simulink library "eltreclib"  (R2017a)
settings: Solver=VariableStepAuto  StartTime=0.0  StopTime=10.0  RelTol=1e-3
undefined symbols (not defined in the file or in its folder): Jr
libraries: powerlib x79
settings Model: Creator=mayartmal  LastModifiedBy=mayartmal

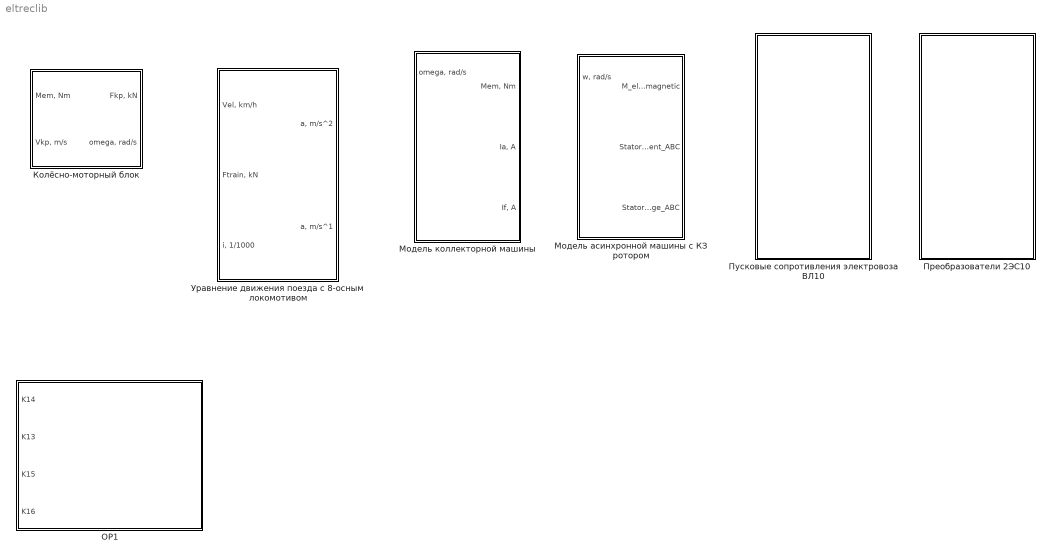
== system eltreclib ==
  OP1 : Subsystem
      mask DialogControl DescTextVar Prompt: Резисторы ослабления поля
  Колёсно-моторный блок : Subsystem  mask{Db=0, mu=0}
      mask prompts: Db "Диаметр бандажа, м"; mu "Передаточное отношение редуктора"
      mask DialogControl DescTextVar Prompt: Здесь можно вписать описание, формулы и другую полезную информацию
  Модель асинхронной машины с КЗ ротором : Subsystem  mask(Модель асинхронной машины){f_nominal=50, Rs=0.0472, ls=0.0003883, Rr=0.0392, lr=0.0005399, Lm=0.011, Zp=2}
      mask prompts: f_nominal "Номинальная частота, Гц"; Rs "Активное сопротивление статора, Ом"; ls "Индуктивность статора, Гн"; Rr "Активное сопротивление ротора, Ом"; lr "Индуктивность ротора, Гн"; Lm "Взаимная индуктивность, Гн"; Zp "Число пар полюсов"
      mask help: Модель учитывает только электрические параметры схемы замещения и не учитывает механику
      mask init:
      | Ls = ls + Lm;
      | Lr = lr + Lm;
      | Kr = Lm / Lr;
      | Ks = Lm / Ls;
      | sigma = 1 - (Lm ^ 2) / (Ls * Lr);
      | w_s = (2 * pi * f_nominal) / Zp;
  Модель коллекторной машины : Subsystem  mask{Rf=0, Lf=0, Ra=0, La=0, Ce=0, Cm=0, A=0, B=0}
      mask prompts: Rf "Активное сопротивление обмотки возбуждения, Ом"; Lf "Индуктивность обмотки возбуждения, Гн"; Ra "Активное сопротивление обмотки якоря, Ом"; La "Индуктивность обмотки якоря, Гн"; Ce "Константа Ce"; Cm "Константа Cm"; A "Коэффициент A"; B "Коэффициент B"
      mask DialogControl DescTextVar Prompt: Здесь можно вписать описание, формулы и другую полезную информацию
  Преобразователи 2ЭС10 : Subsystem
  Пусковые сопротивления электровоза ВЛ10 : Subsystem
  Уравнение движения поезда c 8-осным локомотивом : Subsystem  mask{a0=16, a1=0.176, a2=0.0079, P=112}
      mask prompts: a0 "Коэффициент a0"; a1 "Коэффициент a1"; a2 "Коэффициент a2"; P "Масса поезда, т"
      mask DialogControl DescTextVar Prompt: Здесь можно вписать описание, формулы и другую полезную информацию

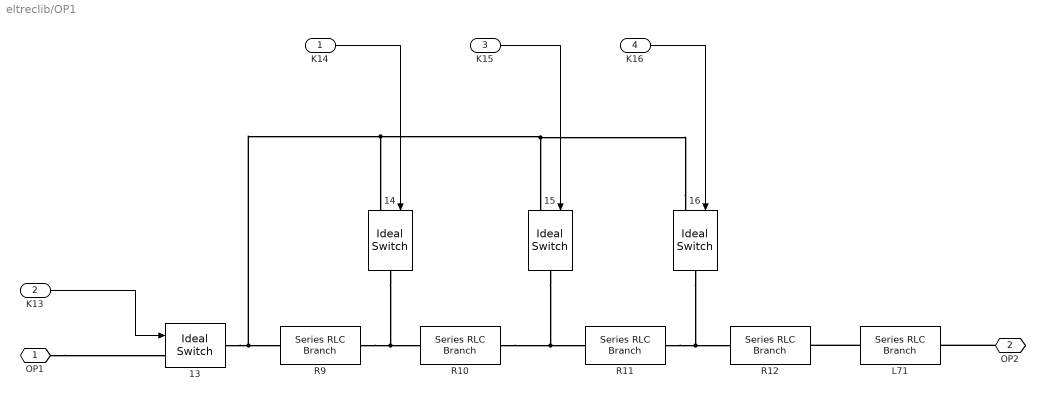
== system eltreclib/OP1 ==
  K14 : Inport
  K13 : Inport  Port=2
  K15 : Inport  Port=3
  K16 : Inport  Port=4
  {13..16} (4 alike) : powerlib/Power Electronics/Ideal Switch  Ron=0.001  Lon=0  IC=0  Rs=1e6  Cs=inf  Measurements=off
  L71 : powerlib/Elements/Series RLC Branch  LConnTagsString=__new0  RConnTagsString=__new0  BranchType=RL  Resistance=0.0236  Inductance=4.5e-3  SetiL0=off  InitialCurrent=0  Capacitance=1e-6  Setx0=off  InitialVoltage=0  Measurements=None
  R10 : powerlib/Elements/Series RLC Branch  LConnTagsString=__new0  RConnTagsString=__new0  BranchType=R  Resistance=0.04  Inductance=1e-3  SetiL0=off  InitialCurrent=0  Capacitance=1e-6  Setx0=off  InitialVoltage=0  Measurements=None
  R11 : powerlib/Elements/Series RLC Branch  LConnTagsString=__new0  RConnTagsString=__new0  BranchType=R  Resistance=0.0222  Inductance=1e-3  SetiL0=off  InitialCurrent=0  Capacitance=1e-6  Setx0=off  InitialVoltage=0  Measurements=None
  R12 : powerlib/Elements/Series RLC Branch  LConnTagsString=__new0  RConnTagsString=__new0  BranchType=R  Resistance=0.01  Inductance=1e-3  SetiL0=off  InitialCurrent=0  Capacitance=1e-6  Setx0=off  InitialVoltage=0  Measurements=None
  R9 : powerlib/Elements/Series RLC Branch  LConnTagsString=__new0  RConnTagsString=__new0  BranchType=R  Resistance=0.1407  Inductance=1e-3  SetiL0=off  InitialCurrent=0  Capacitance=1e-6  Setx0=off  InitialVoltage=0  Measurements=None
  OP1 : PMIOPort  Port=1  Side=Right
  OP2 : PMIOPort  Port=2  Side=Right
  wires:
  K16/1 -> 16/1
  K15/1 -> 15/1
  K13/1 -> 13/1
  K14/1 -> 14/1
  connections:
  OP2/RConn1 -- L71/RConn1
  L71/LConn1 -- R12/RConn1
  OP1/RConn1 -- 13/LConn1
  16/LConn1 -- 14/LConn1 -- 13/RConn1 -- R9/LConn1 -- 15/LConn1
  16/RConn1 -- R11/RConn1 -- R12/LConn1
  15/RConn1 -- R10/RConn1 -- R11/LConn1
  14/RConn1 -- R9/RConn1 -- R10/LConn1

== system eltreclib/Колёсно-моторный блок ==
  "Mem, Nm" : Inport
  "Vkp, m/s" : Inport  Port=2
  Gain : Gain  Gain=mu
  Gain1 : Gain  Gain=2/Db
  Gain2 : Gain  Gain=0.001
  Gain5 : Gain  Gain=2/Db
  Gain6 : Gain  Gain=mu
  "Fkp, kN" : Outport
  "omega, rad/s" : Outport  Port=2
  wires:
  Gain/1 -> Gain1/1  "Mkp, Nm"
  "Mem, Nm"/1 -> Gain/1
  Gain1/1 -> Gain2/1  "Fkp, N"
  Gain5/1 -> Gain6/1
  "Vkp, m/s"/1 -> Gain5/1
  Gain6/1 -> "omega, rad/s"/1
  Gain2/1 -> "Fkp, kN"/1

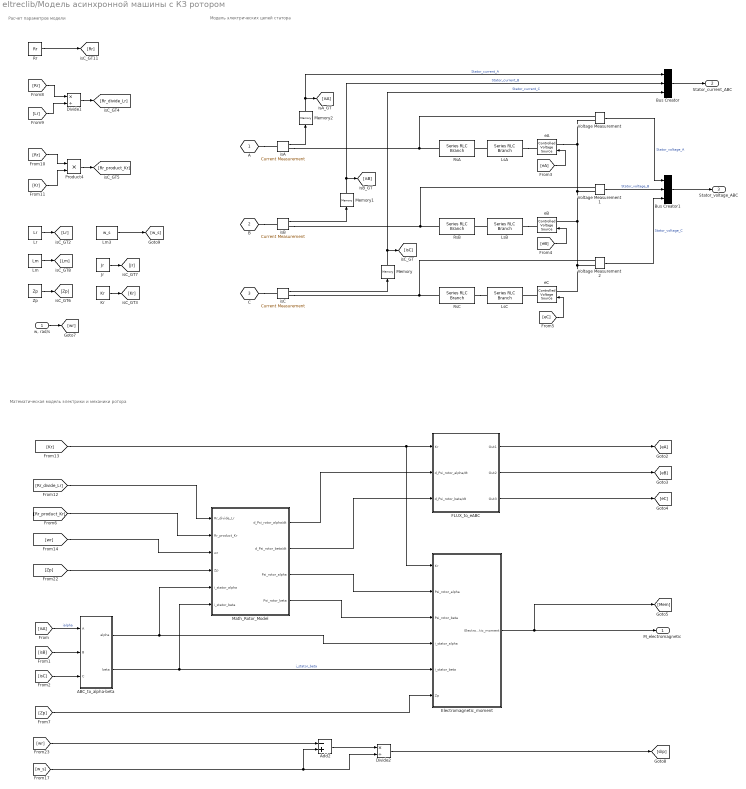
== system eltreclib/Модель асинхронной машины с КЗ ротором ==
  note: Математическая модель электрики и механики ротора
  note: Расчет параметров модели
  note: Модель электрических цепей статора
  "w, rad/s" : Inport
  ABC_to_alpha-beta : Subsystem
  Add2 : Sum  Inputs=-+
  Bus Creator : BusCreator  Inputs=3
  Bus Creator1 : BusCreator  Inputs=3
  Divide1 : Product  Inputs=*/
  Divide2 : Product  Inputs=*/
  "Electromagnetic_moment " : Subsystem
  FLUX_to_eABC : Subsystem
  Jr : Constant  Value=Jr
  Kr : Constant  Value=Kr
  Lm : Constant  Value=Lm
  Lm3 : Constant  Value=w_s
  Lr : Constant  Value=Lr
  LsA : powerlib/Elements/Series RLC Branch  LConnTagsString=__new0  RConnTagsString=__new0  BranchType=L  Resistance=Rs  Inductance=Ls * sigma  SetiL0=off  InitialCurrent=0  Capacitance=1e-6  Setx0=off  InitialVoltage=0  Measurements=None
  LsB : powerlib/Elements/Series RLC Branch  LConnTagsString=__new0  RConnTagsString=__new0  BranchType=L  Resistance=Rs  Inductance=Ls * sigma  SetiL0=off  InitialCurrent=0  Capacitance=1e-6  Setx0=off  InitialVoltage=0  Measurements=None
  LsC : powerlib/Elements/Series RLC Branch  LConnTagsString=__new0  RConnTagsString=__new0  BranchType=L  Resistance=Rs  Inductance=Ls * sigma  SetiL0=off  InitialCurrent=0  Capacitance=1e-6  Setx0=off  InitialVoltage=0  Measurements=None
  Math_Rotor_Model : Subsystem
  Memory : Memory
  Memory1 : Memory
  Memory2 : Memory
  Product4 : Product
  Rr : Constant  Value=Rr
  RsA : powerlib/Elements/Series RLC Branch  LConnTagsString=__new0  RConnTagsString=__new0  BranchType=R  Resistance=Rs  Inductance=1e-3  SetiL0=off  InitialCurrent=0  Capacitance=1e-6  Setx0=off  InitialVoltage=0  Measurements=None
  RsB : powerlib/Elements/Series RLC Branch  LConnTagsString=__new0  RConnTagsString=__new0  BranchType=R  Resistance=Rs  Inductance=1e-3  SetiL0=off  InitialCurrent=0  Capacitance=1e-6  Setx0=off  InitialVoltage=0  Measurements=None
  RsC : powerlib/Elements/Series RLC Branch  LConnTagsString=__new0  RConnTagsString=__new0  BranchType=R  Resistance=Rs  Inductance=1e-3  SetiL0=off  InitialCurrent=0  Capacitance=1e-6  Setx0=off  InitialVoltage=0  Measurements=None
  Voltage Measurement : powerlib/Measurements/Voltage Measurement  PhasorSimulation=off  OutputType=Complex  PSBequivalent=0
  Voltage Measurement1 : powerlib/Measurements/Voltage Measurement  PhasorSimulation=off  OutputType=Complex  PSBequivalent=0
  Voltage Measurement2 : powerlib/Measurements/Voltage Measurement  PhasorSimulation=off  OutputType=Complex  PSBequivalent=0
  Zp : Constant  Value=Zp
  eA : powerlib/Electrical Sources/Controlled Voltage Source  Initialize=on  Source_Type=AC  Amplitude=0  Phase=0  Frequency=0  Measurements=None
  eB : powerlib/Electrical Sources/Controlled Voltage Source  Initialize=on  Source_Type=AC  Amplitude=0  Phase=0  Frequency=0  Measurements=None
  eC : powerlib/Electrical Sources/Controlled Voltage Source  Initialize=on  Source_Type=AC  Amplitude=0  Phase=0  Frequency=0  Measurements=None
  isA : powerlib/Measurements/Current Measurement  PhasorSimulation=off  OutputType=Complex  PSBequivalent=0
  isB : powerlib/Measurements/Current Measurement  PhasorSimulation=off  OutputType=Complex  PSBequivalent=0
  isC : powerlib/Measurements/Current Measurement  PhasorSimulation=off  OutputType=Complex  PSBequivalent=0
  A : PMIOPort  Tag=PMCPort  Port=1  Side=Left
  B : PMIOPort  Tag=PMCPort  Port=2  Side=Left
  C : PMIOPort  Tag=PMCPort  Port=3  Side=Left
  M_electromagnetic : Outport
  Stator_current_ABC : Outport  Port=2
  Stator_voltage_ABC : Outport  Port=3
  wires:
  "w, rad/s"/1 -> [wr]
  [Lr] -> Divide1/2
  Divide1/1 -> [Rr_divide_Lr]
  Zp/1 -> [Zp]
  Jr/1 -> [Jr]
  Lr/1 -> [Lr]
  [Rr] -> Divide1/1
  [eB] -> eB/1
  [eA] -> eA/1
  [eC] -> eC/1
  [Rr] -> Product4/1
  [Kr] -> Product4/2
  Product4/1 -> [Rr_product_Kr]
  [isA] -> ABC_to_alpha-beta/1(A)  "ialpha"
  Lm/1 -> [Lm]
  Kr/1 -> [Kr]
  isC/1 -> Memory/1
  isB/1 -> Memory1/1
  isA/1 -> Memory2/1
  Memory/1 -> Bus Creator/3, [isC]  "Stator_current_C"
  Memory1/1 -> Bus Creator/2, [isB]  "Stator_current_B"
  Memory2/1 -> Bus Creator/1, [isA]  "Stator_current_A"
  ABC_to_alpha-beta/2(beta) -> Math_Rotor_Model/6(i_stator_beta), "Electromagnetic_moment "/5(i_stator_beta)  "i_stator_beta"
  [isB] -> ABC_to_alpha-beta/2(B)
  [isC] -> ABC_to_alpha-beta/3(C)
  ABC_to_alpha-beta/1(alpha) -> Math_Rotor_Model/5(i_stator_alpha), "Electromagnetic_moment "/4(i_stator_alpha)
  Bus Creator/1 -> Stator_current_ABC/1
  "Electromagnetic_moment "/1(Electromagnetic_moment) -> M_electromagnetic/1, [Mem]
  [Kr] -> "Electromagnetic_moment "/1(Kr), FLUX_to_eABC/1(Kr)
  FLUX_to_eABC/1(Out1) -> [eA]
  FLUX_to_eABC/2(Out2) -> [eB]
  FLUX_to_eABC/3(Out3) -> [eC]
  [Rr_divide_Lr] -> Math_Rotor_Model/1(Rr_divide_Lr)
  [Rr_product_Kr] -> Math_Rotor_Model/2(Rr_product_Kr)
  Math_Rotor_Model/1(d_Psi_rotor_alpha/dt) -> FLUX_to_eABC/2(d_Psi_rotor_alpha/dt)
  Math_Rotor_Model/2(d_Psi_rotor_beta/dt) -> FLUX_to_eABC/3(d_Psi_rotor_beta/dt)
  Math_Rotor_Model/4(Psi_rotor_beta) -> "Electromagnetic_moment "/3(Psi_rotor_beta)
  Math_Rotor_Model/3(Psi_rotor_alpha) -> "Electromagnetic_moment "/2(Psi_rotor_alpha)
  [Zp] -> "Electromagnetic_moment "/6(Zp)
  [wr] -> Math_Rotor_Model/3(wr)
  [Zp] -> Math_Rotor_Model/4(Zp)
  Rr/1 -> [Rr]
  Lm3/1 -> [w_s]
  [w_s] -> Add2/2, Divide2/2
  [wr] -> Add2/1
  Add2/1 -> Divide2/1
  Divide2/1 -> [slip]
  Voltage Measurement/1 -> Bus Creator1/1  "Stator_voltage_A"
  Voltage Measurement1/1 -> Bus Creator1/2  "Stator_voltage_B"
  Voltage Measurement2/1 -> Bus Creator1/3  "Stator_voltage_C"
  Bus Creator1/1 -> Stator_voltage_ABC/1
  connections:
  LsB/LConn1 -- RsB/RConn1
  RsC/RConn1 -- LsC/LConn1
  LsA/LConn1 -- RsA/RConn1
  C/RConn1 -- isC/LConn1
  isC/RConn1 -- Voltage Measurement2/LConn1 -- RsC/LConn1
  B/RConn1 -- isB/LConn1
  isB/RConn1 -- Voltage Measurement1/LConn1 -- RsB/LConn1
  A/RConn1 -- isA/LConn1
  isA/RConn1 -- Voltage Measurement/LConn1 -- RsA/LConn1
  eC/RConn1 -- LsC/RConn1
  LsA/RConn1 -- eA/RConn1
  eA/LConn1 -- Voltage Measurement/LConn2 -- Voltage Measurement1/LConn2 -- eB/LConn1 -- Voltage Measurement2/LConn2 -- eC/LConn1
  LsB/RConn1 -- eB/RConn1

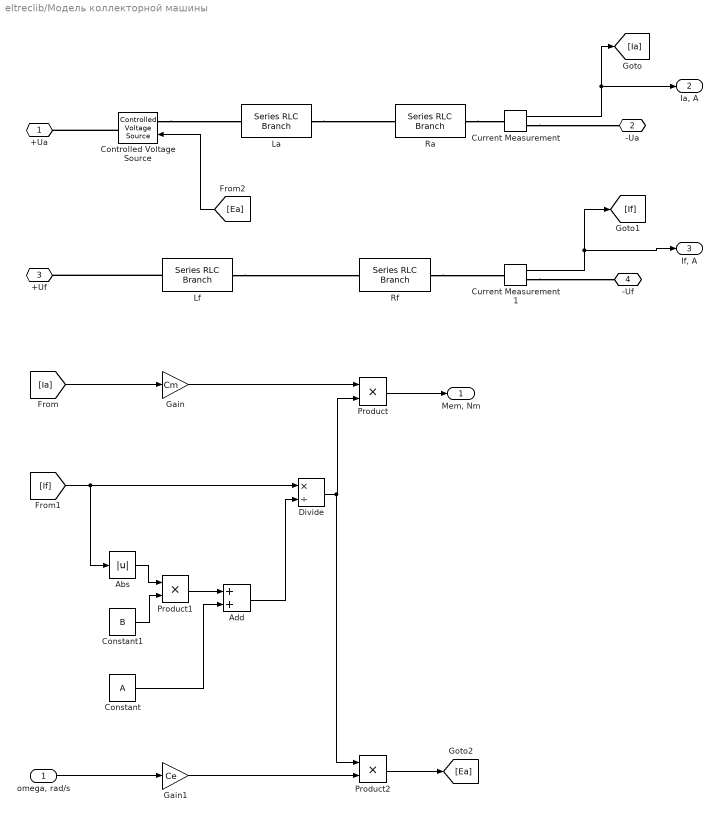
== system eltreclib/Модель коллекторной машины ==
  "omega, rad/s" : Inport
  Abs : Abs
  Add : Sum
  Constant : Constant  Value=A
  Constant1 : Constant  Value=B
  Controlled Voltage Source : powerlib/Electrical Sources/Controlled Voltage Source  Initialize=on  Source_Type=AC  Amplitude=0  Phase=0  Frequency=0  Measurements=None
  Current Measurement : powerlib/Measurements/Current Measurement  PhasorSimulation=off  OutputType=Complex  PSBequivalent=0
  Current Measurement1 : powerlib/Measurements/Current Measurement  PhasorSimulation=off  OutputType=Complex  PSBequivalent=0
  Divide : Product  Inputs=*/
  Gain : Gain  Gain=Cm
  Gain1 : Gain  Gain=Ce
  La : powerlib/Elements/Series RLC Branch  LConnTagsString=__new0  RConnTagsString=__new0  BranchType=L  Resistance=1  Inductance=La  SetiL0=off  InitialCurrent=0  Capacitance=1e-6  Setx0=off  InitialVoltage=0  Measurements=None
  Lf : powerlib/Elements/Series RLC Branch  LConnTagsString=__new0  RConnTagsString=__new0  BranchType=L  Resistance=1  Inductance=Lf  SetiL0=off  InitialCurrent=0  Capacitance=1e-6  Setx0=off  InitialVoltage=0  Measurements=None
  Product : Product
  Product1 : Product
  Product2 : Product
  Ra : powerlib/Elements/Series RLC Branch  LConnTagsString=__new0  RConnTagsString=__new0  BranchType=R  Resistance=Ra  Inductance=1e-3  SetiL0=off  InitialCurrent=0  Capacitance=1e-6  Setx0=off  InitialVoltage=0  Measurements=None
  Rf : powerlib/Elements/Series RLC Branch  LConnTagsString=__new0  RConnTagsString=__new0  BranchType=R  Resistance=Rf  Inductance=1e-3  SetiL0=off  InitialCurrent=0  Capacitance=1e-6  Setx0=off  InitialVoltage=0  Measurements=None
  +Ua : PMIOPort  Port=1  Side=Left
  -Ua : PMIOPort  Port=2  Side=Left
  +Uf : PMIOPort  Port=3  Side=Left
  -Uf : PMIOPort  Port=4  Side=Left
  "Mem, Nm" : Outport
  "Ia, A" : Outport  Port=2
  "If, A" : Outport  Port=3
  wires:
  Product/1 -> "Mem, Nm"/1
  Product2/1 -> [Ea]
  Gain1/1 -> Product2/2
  "omega, rad/s"/1 -> Gain1/1
  Divide/1 -> Product/2, Product2/1
  Add/1 -> Divide/2
  Product1/1 -> Add/1
  Constant/1 -> Add/2
  Constant1/1 -> Product1/2
  Abs/1 -> Product1/1
  [If] -> Abs/1, Divide/1
  Gain/1 -> Product/1
  [Ia] -> Gain/1
  Current Measurement1/1 -> [If], "If, A"/1
  Current Measurement/1 -> "Ia, A"/1, [Ia]
  [Ea] -> Controlled Voltage Source/1
  connections:
  Current Measurement1/RConn1 -- -Uf/RConn1
  Rf/RConn1 -- Current Measurement1/LConn1
  Current Measurement/RConn1 -- -Ua/RConn1
  Ra/RConn1 -- Current Measurement/LConn1
  Controlled Voltage Source/LConn1 -- La/LConn1
  Lf/RConn1 -- Rf/LConn1
  Controlled Voltage Source/RConn1 -- +Ua/RConn1
  Lf/LConn1 -- +Uf/RConn1
  La/RConn1 -- Ra/LConn1

== system eltreclib/Преобразователи 2ЭС10 ==
  Bogie electric drive : Subsystem
      mask DialogControl DescGroupVar Prompt: Модель электропривода тележки
      mask DialogControl DescTextVar Prompt: Подсистема включает в себя набор электрооборудования и преобразователей, питающих двигатели одной тележки

== system eltreclib/Пусковые сопротивления электровоза ВЛ10 ==
  Блок пусковых сопротивлений I : Subsystem
      mask DialogControl DescGroupVar Prompt: Блок пусковых сопротивлений I
      mask DialogControl DescTextVar Prompt: Моделирует схему блока пусковых сопротивлений, собранного из резисторов R1=3.15 Ом, R2=1.47 Ом, R3=1.2 Ом
  Блок пусковых сопротивлений II : Subsystem
      mask DialogControl DescGroupVar Prompt: Блок пусковых сопротивлений II
      mask DialogControl DescTextVar Prompt: Моделирует схему блока пусковых сопротивлений, собранного из резисторов R5=4.725 Ом, R6=0.841 Ом, R7=1.312 Ом
  Блок пусковых сопротивлений III : Subsystem
      mask DialogControl DescGroupVar Prompt: Блок пусковых сопротивлений III
      mask DialogControl DescTextVar Prompt: Моделирует схему блока пусковых сопротивлений, собранного из резисторов R23=1.9425 Ом, R24=0.8 Ом, R25=0.61 Ом
  Блок пусковых сопротивлений IV : Subsystem
      mask DialogControl DescGroupVar Prompt: Блок пусковых сопротивлений IV
      mask DialogControl DescTextVar Prompt: Моделирует схему блока пусковых сопротивлений, собранного из резисторов R27=5.775 Ом, R28=0.595 Ом, R29=0.4315 Ом

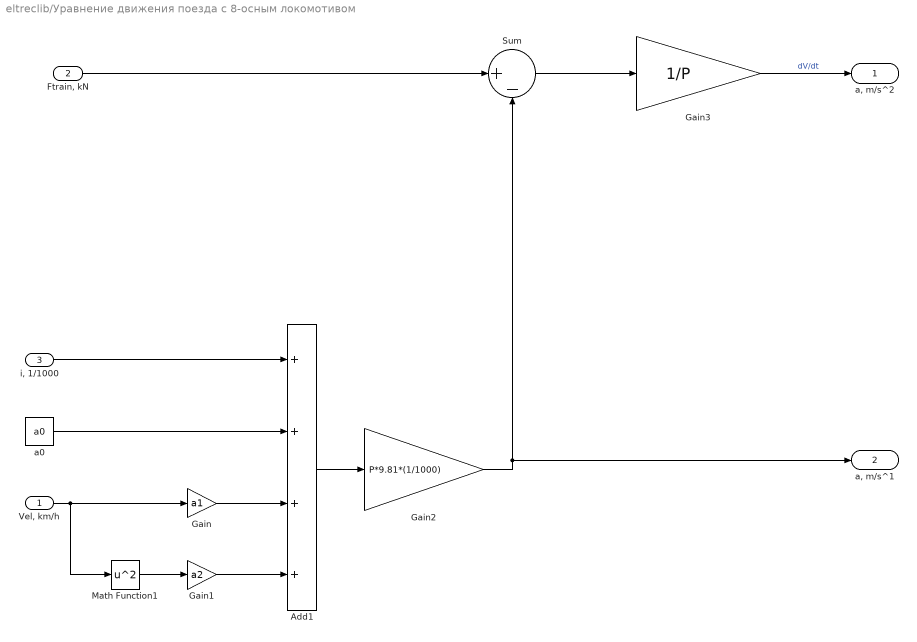
== system eltreclib/Уравнение движения поезда c 8-осным локомотивом ==
  "Vel, km/h" : Inport
  "Ftrain, kN" : Inport  Port=2
  "i, 1/1000" : Inport  Port=3
  Add1 : Sum  Inputs=++++
  Gain : Gain  Gain=a1
  Gain1 : Gain  Gain=a2
  Gain2 : Gain  Gain=P*9.81*(1/1000)
  Gain3 : Gain  Gain=1/P
  Math Function1 : Math  Operator=square  SaturateOnIntegerOverflow=on
  Sum : Sum  Inputs=|+-
  a0 : Constant  Value=a0
  "a, m/s^2" : Outport
  "a, m/s^1" : Outport  Port=2
  wires:
  "Ftrain, kN"/1 -> Sum/1
  "Vel, km/h"/1 -> Math Function1/1, Gain/1
  a0/1 -> Add1/2
  Gain/1 -> Add1/3
  Sum/1 -> Gain3/1
  Gain3/1 -> "a, m/s^2"/1  "dV/dt"
  Gain2/1 -> "a, m/s^1"/1, Sum/2
  Math Function1/1 -> Gain1/1
  Gain1/1 -> Add1/4
  Add1/1 -> Gain2/1
  "i, 1/1000"/1 -> Add1/1

== system eltreclib/Модель асинхронной машины с КЗ ротором/ABC_to_alpha-beta ==
  A : Inport
  B : Inport  Port=2
  C : Inport  Port=3
  2 : Gain  Gain=1/sqrt(3)
  3 : Gain  Gain=1/sqrt(3)
  Add : Sum  Inputs=+-
  alpha : Outport
  beta : Outport  Port=2
  wires:
  3/1 -> Add/1
  B/1 -> 3/1
  C/1 -> 2/1
  Add/1 -> beta/1  "ibeta"
  2/1 -> Add/2
  A/1 -> alpha/1

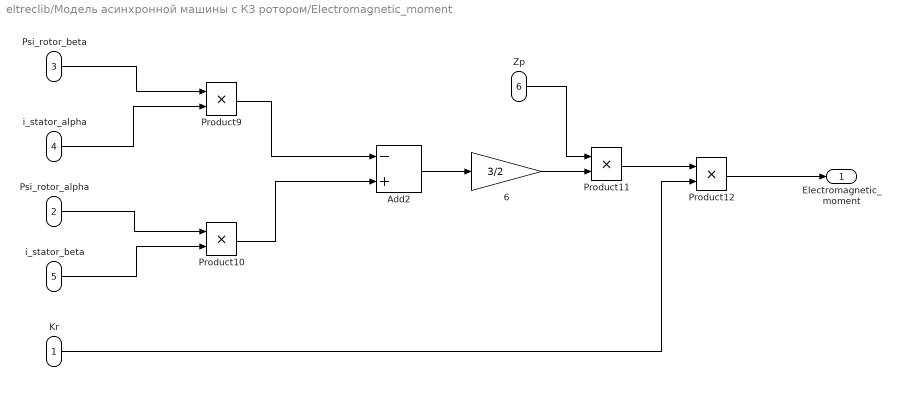
== system eltreclib/Модель асинхронной машины с КЗ ротором/Electromagnetic_moment  ==
  Kr : Inport
  Psi_rotor_alpha : Inport  Port=2
  Psi_rotor_beta : Inport  Port=3
  i_stator_alpha : Inport  Port=4
  i_stator_beta : Inport  Port=5
  Zp : Inport  Port=6
  6 : Gain  Gain=3/2
  Add2 : Sum  Inputs=-+
  Product{9..12} (4 alike) : Product
  Electromagnetic_moment : Outport
  wires:
  Product11/1 -> Product12/1
  Kr/1 -> Product12/2
  Product10/1 -> Add2/2
  Product9/1 -> Add2/1
  Product12/1 -> Electromagnetic_moment/1
  6/1 -> Product11/2
  Zp/1 -> Product11/1
  Add2/1 -> 6/1
  i_stator_alpha/1 -> Product9/2
  Psi_rotor_alpha/1 -> Product10/1
  Psi_rotor_beta/1 -> Product9/1
  i_stator_beta/1 -> Product10/2

== system eltreclib/Модель асинхронной машины с КЗ ротором/FLUX_to_eABC ==
  Kr : Inport
  d_Psi_rotor_alpha/dt : Inport  Port=2
  d_Psi_rotor_beta/dt : Inport  Port=3
  1 : Gain  Gain=1/2
  5 : Gain  Gain=sqrt(3)/2
  Add5 : Sum  Inputs=-+
  Add6 : Sum  Inputs=--
  Product3 : Product
  Product6 : Product
  Out1 : Outport
  Out2 : Outport  Port=2
  Out3 : Outport  Port=3
  wires:
  Product6/1 -> 5/1
  1/1 -> Add5/1, Add6/1
  5/1 -> Add5/2, Add6/2
  Add6/1 -> Out3/1
  Kr/1 -> Product6/1, Product3/1
  Product3/1 -> Out1/1, 1/1
  Add5/1 -> Out2/1
  d_Psi_rotor_alpha/dt/1 -> Product3/2
  d_Psi_rotor_beta/dt/1 -> Product6/2

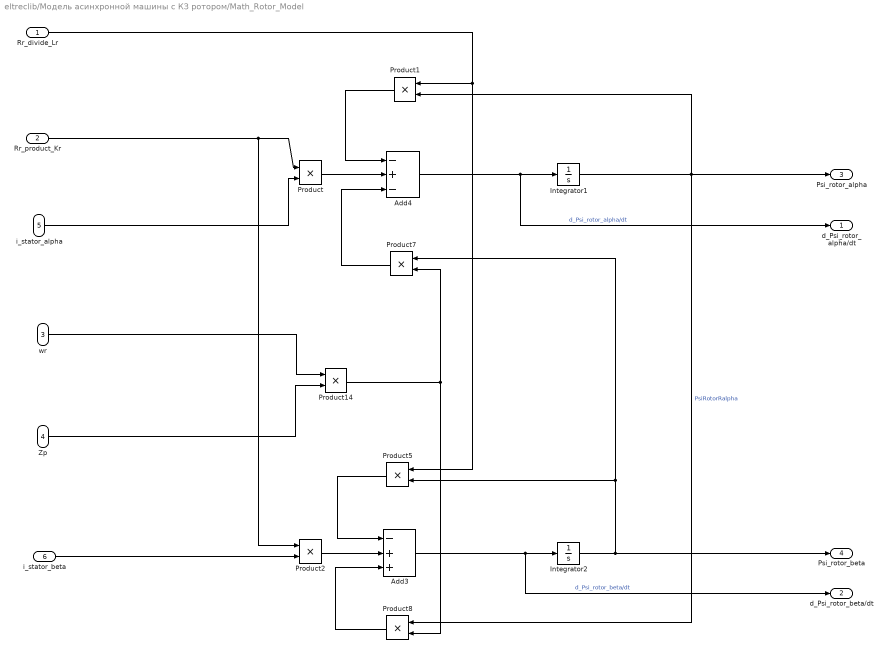
== system eltreclib/Модель асинхронной машины с КЗ ротором/Math_Rotor_Model ==
  Rr_divide_Lr : Inport
  Rr_product_Kr : Inport  Port=2
  wr : Inport  Port=3
  Zp : Inport  Port=4
  i_stator_alpha : Inport  Port=5
  i_stator_beta : Inport  Port=6
  Add3 : Sum  Inputs=-++
  Add4 : Sum  Inputs=-+-
  Integrator1 : Integrator
  Integrator2 : Integrator
  Product{,1..2,5,7..8,14} (7 alike) : Product
  d_Psi_rotor_alpha/dt : Outport
  d_Psi_rotor_beta/dt : Outport  Port=2
  Psi_rotor_alpha : Outport  Port=3
  Psi_rotor_beta : Outport  Port=4
  wires:
  Zp/1 -> Product14/2
  Product14/1 -> Product7/2, Product8/2
  Product1/1 -> Add4/1
  Product7/1 -> Add4/3
  Rr_product_Kr/1 -> Product/1, Product2/1
  Product5/1 -> Add3/1
  Integrator1/1 -> Product1/2, Product8/1, Psi_rotor_alpha/1  "PsiRotorRalpha"
  wr/1 -> Product14/1
  Product/1 -> Add4/2
  Product2/1 -> Add3/2
  Product8/1 -> Add3/3
  Rr_divide_Lr/1 -> Product1/1, Product5/1
  Add3/1 -> d_Psi_rotor_beta/dt/1, Integrator2/1  "d_Psi_rotor_beta/dt"
  Integrator2/1 -> Product5/2, Product7/1, Psi_rotor_beta/1
  Add4/1 -> d_Psi_rotor_alpha/dt/1, Integrator1/1  "d_Psi_rotor_alpha/dt"
  i_stator_beta/1 -> Product2/2
  i_stator_alpha/1 -> Product/2

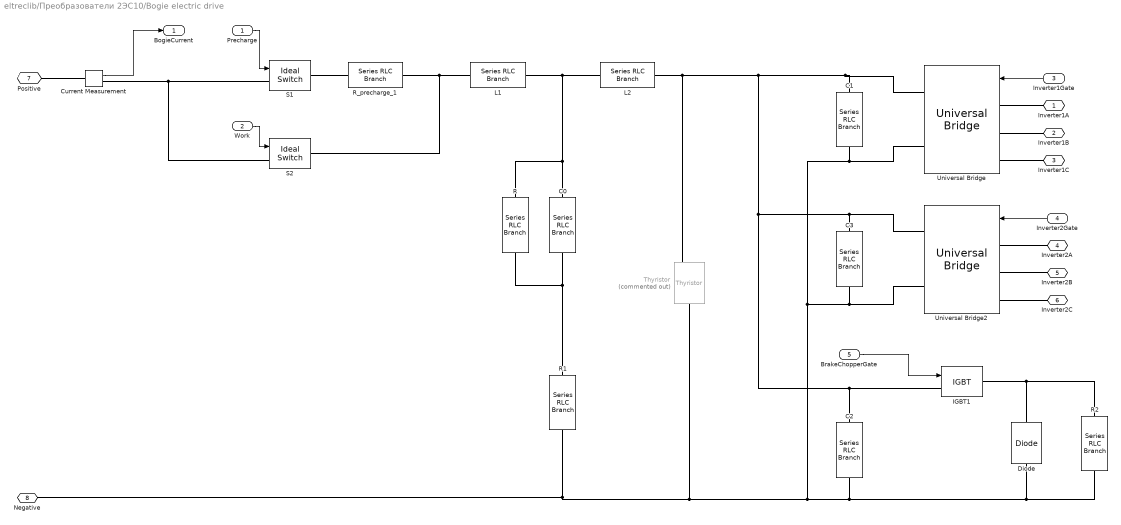
== system eltreclib/Преобразователи 2ЭС10/Bogie electric drive ==
  Precharge : Inport
  Work : Inport  Port=2
  Inverter1Gate : Inport  Port=3
  Inverter2Gate : Inport  Port=4
  BrakeChopperGate : Inport  Port=5
  C0 : powerlib/Elements/Series RLC Branch  LConnTagsString=__new0  RConnTagsString=__new0  BranchType=C  Resistance=112  Inductance=39e-3  SetiL0=off  InitialCurrent=0  Capacitance=7.56e-3  Setx0=off  InitialVoltage=0  Measurements=None
  C1 : powerlib/Elements/Series RLC Branch  LConnTagsString=__new0  RConnTagsString=__new0  BranchType=C  Resistance=112  Inductance=39e-3  SetiL0=off  InitialCurrent=0  Capacitance=2e-3  Setx0=off  InitialVoltage=0  Measurements=None
  C2 : powerlib/Elements/Series RLC Branch  LConnTagsString=__new0  RConnTagsString=__new0  BranchType=C  Resistance=112  Inductance=39e-3  SetiL0=off  InitialCurrent=0  Capacitance=7.56e-3  Setx0=off  InitialVoltage=0  Measurements=None
  C3 : powerlib/Elements/Series RLC Branch  LConnTagsString=__new0  RConnTagsString=__new0  BranchType=C  Resistance=112  Inductance=39e-3  SetiL0=off  InitialCurrent=0  Capacitance=2e-3  Setx0=off  InitialVoltage=0  Measurements=None
  Current Measurement : powerlib/Measurements/Current Measurement  PhasorSimulation=off  OutputType=Complex  PSBequivalent=0
  Diode : powerlib/Power Electronics/Diode  Ron=0.001  Lon=0  Vf=0.8  IC=0  UseSnubber=0  Rs=500  Cs=250e-9  Measurements=off
  IGBT1 : powerlib/Power Electronics/IGBT  Ron=0.001  Lon=0  Vf=1  Tf=1e-6  Tt=2e-6  IC=0  Rs=1e5  Cs=inf  Measurements=off
  L1 : powerlib/Elements/Series RLC Branch  LConnTagsString=__new0  RConnTagsString=__new0  BranchType=L  Resistance=112  Inductance=39e-3  SetiL0=off  InitialCurrent=0  Capacitance=1e-6  Setx0=off  InitialVoltage=0  Measurements=None
  L2 : powerlib/Elements/Series RLC Branch  LConnTagsString=__new0  RConnTagsString=__new0  BranchType=L  Resistance=112  Inductance=3.15e-3  SetiL0=off  InitialCurrent=0  Capacitance=1e-6  Setx0=off  InitialVoltage=0  Measurements=None
  R : powerlib/Elements/Series RLC Branch  LConnTagsString=__new0  RConnTagsString=__new0  BranchType=R  Resistance=1e6  Inductance=1e-3  SetiL0=off  InitialCurrent=0  Capacitance=1e-6  Setx0=off  InitialVoltage=0  Measurements=None
  R1 : powerlib/Elements/Series RLC Branch  LConnTagsString=__new0  RConnTagsString=__new0  BranchType=R  Resistance=1  Inductance=1e-3  SetiL0=off  InitialCurrent=0  Capacitance=1e-6  Setx0=off  InitialVoltage=0  Measurements=None
  R2 : powerlib/Elements/Series RLC Branch  LConnTagsString=__new0  RConnTagsString=__new0  BranchType=R  Resistance=5  Inductance=1e-3  SetiL0=off  InitialCurrent=0  Capacitance=1e-6  Setx0=off  InitialVoltage=0  Measurements=None
  R_precharge_1 : powerlib/Elements/Series RLC Branch  LConnTagsString=__new0  RConnTagsString=__new0  BranchType=R  Resistance=112  Inductance=1e-3  SetiL0=off  InitialCurrent=0  Capacitance=1e-6  Setx0=off  InitialVoltage=0  Measurements=None
  S1 : powerlib/Power Electronics/Ideal Switch  Ron=0.001  Lon=0  IC=0  Rs=1e6  Cs=inf  Measurements=off
  S2 : powerlib/Power Electronics/Ideal Switch  Ron=0.001  Lon=0  IC=0  Rs=1e6  Cs=inf  Measurements=off
  Thyristor : powerlib/Power Electronics/Thyristor  Commented=on  Ron=0.001  Lon=0  Vf=0.8  IC=0  Rs=500  Cs=250e-9  Measurements=off
  Universal Bridge : powerlib/Power Electronics/Universal Bridge  Arms=3  SnubberResistance=1e5  SnubberCapacitance=inf  Device=IGBT / Diodes  Ron=1e-3  Lon=0  ForwardVoltages="[  0  0  ]"  ForwardVoltage=0  GTOparameters=[ 10e-6 , 20e-6 ]  IGBTparameters=[ 1e-6 , 2e-6 ]  Measurements=None  Measurements_2=None  converterType=Rectifier
  Universal Bridge2 : powerlib/Power Electronics/Universal Bridge  Arms=3  SnubberResistance=1e5  SnubberCapacitance=inf  Device=IGBT / Diodes  Ron=1e-3  Lon=0  ForwardVoltages="[  0  0  ]"  ForwardVoltage=0  GTOparameters=[ 10e-6 , 20e-6 ]  IGBTparameters=[ 1e-6 , 2e-6 ]  Measurements=None  Measurements_2=None  converterType=Rectifier
  Inverter1A : PMIOPort  Port=1  Side=Right
  Inverter1B : PMIOPort  Port=2  Side=Right
  Inverter1C : PMIOPort  Port=3  Side=Right
  Inverter2A : PMIOPort  Port=4  Side=Right
  Inverter2B : PMIOPort  Port=5  Side=Right
  Inverter2C : PMIOPort  Port=6  Side=Right
  Positive : PMIOPort  Port=7  Side=Left
  Negative : PMIOPort  Port=8  Side=Left
  BogieCurrent : Outport
  wires:
  Inverter2Gate/1 -> Universal Bridge2/1
  Inverter1Gate/1 -> Universal Bridge/1
  Work/1 -> S2/1
  Precharge/1 -> S1/1
  BrakeChopperGate/1 -> IGBT1/1
  Current Measurement/1 -> BogieCurrent/1
  connections:
  IGBT1/LConn1 -- C2/LConn1 -- C1/LConn1 -- Universal Bridge/RConn1 -- Thyristor/LConn1 -- L2/RConn1 -- C3/LConn1 -- Universal Bridge2/RConn1
  Universal Bridge2/LConn2 -- Inverter2B/RConn1
  Universal Bridge2/LConn3 -- Inverter2C/RConn1
  Universal Bridge/LConn1 -- Inverter1A/RConn1
  Universal Bridge2/LConn1 -- Inverter2A/RConn1
  Universal Bridge/LConn3 -- Inverter1C/RConn1
  Current Measurement/LConn1 -- Positive/RConn1
  Inverter1B/RConn1 -- Universal Bridge/LConn2
  Diode/RConn1 -- R2/LConn1 -- IGBT1/RConn1
  R1/LConn1 -- C0/RConn1 -- R/RConn1
  L1/RConn1 -- C0/LConn1 -- R/LConn1 -- L2/LConn1
  L1/LConn1 -- S2/RConn1 -- R_precharge_1/RConn1
  R1/RConn1 -- Negative/RConn1 -- C1/RConn1 -- Universal Bridge/RConn2 -- C3/RConn1 -- Universal Bridge2/RConn2 -- C2/RConn1 -- Diode/LConn1 -- R2/RConn1 -- Thyristor/RConn1
  R_precharge_1/LConn1 -- S1/RConn1
  S1/LConn1 -- Current Measurement/RConn1 -- S2/LConn1

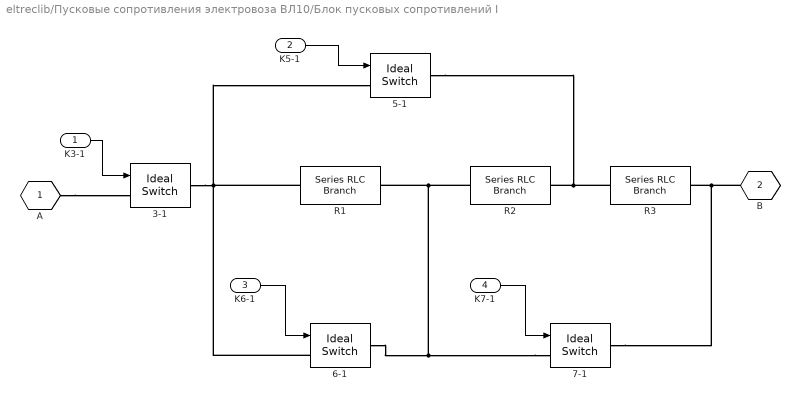
== system eltreclib/Пусковые сопротивления электровоза ВЛ10/Блок пусковых сопротивлений I ==
  K3-1 : Inport
  K5-1 : Inport  Port=2
  K6-1 : Inport  Port=3
  K7-1 : Inport  Port=4
  3-1 : powerlib/Power Electronics/Ideal Switch  Ron=0.001  Lon=0  IC=0  Rs=1e6  Cs=inf  Measurements=off
  5-1 : powerlib/Power Electronics/Ideal Switch  Ron=0.001  Lon=0  IC=0  Rs=1e6  Cs=inf  Measurements=off
  6-1 : powerlib/Power Electronics/Ideal Switch  Ron=0.001  Lon=0  IC=0  Rs=1e6  Cs=inf  Measurements=off
  7-1 : powerlib/Power Electronics/Ideal Switch  Ron=0.001  Lon=0  IC=0  Rs=1e6  Cs=inf  Measurements=off
  R1 : powerlib/Elements/Series RLC Branch  LConnTagsString=__new0  RConnTagsString=__new0  BranchType=R  Resistance=3.15  Inductance=1e-3  SetiL0=off  InitialCurrent=0  Capacitance=1e-6  Setx0=off  InitialVoltage=0  Measurements=None
  R2 : powerlib/Elements/Series RLC Branch  LConnTagsString=__new0  RConnTagsString=__new0  BranchType=R  Resistance=1.47  Inductance=1e-3  SetiL0=off  InitialCurrent=0  Capacitance=1e-6  Setx0=off  InitialVoltage=0  Measurements=None
  R3 : powerlib/Elements/Series RLC Branch  LConnTagsString=__new0  RConnTagsString=__new0  BranchType=R  Resistance=1.2  Inductance=1e-3  SetiL0=off  InitialCurrent=0  Capacitance=1e-6  Setx0=off  InitialVoltage=0  Measurements=None
  A : PMIOPort  Tag=PMCPort  Port=1  Side=Left
  B : PMIOPort  Tag=PMCPort  Port=2  Side=Right
  wires:
  K6-1/1 -> 6-1/1
  K3-1/1 -> 3-1/1
  K7-1/1 -> 7-1/1
  K5-1/1 -> 5-1/1
  connections:
  A/RConn1 -- 3-1/LConn1
  6-1/LConn1 -- R1/LConn1 -- 3-1/RConn1 -- 5-1/LConn1
  R3/LConn1 -- R2/RConn1 -- 5-1/RConn1
  B/RConn1 -- R3/RConn1 -- 7-1/RConn1
  7-1/LConn1 -- 6-1/RConn1 -- R2/LConn1 -- R1/RConn1

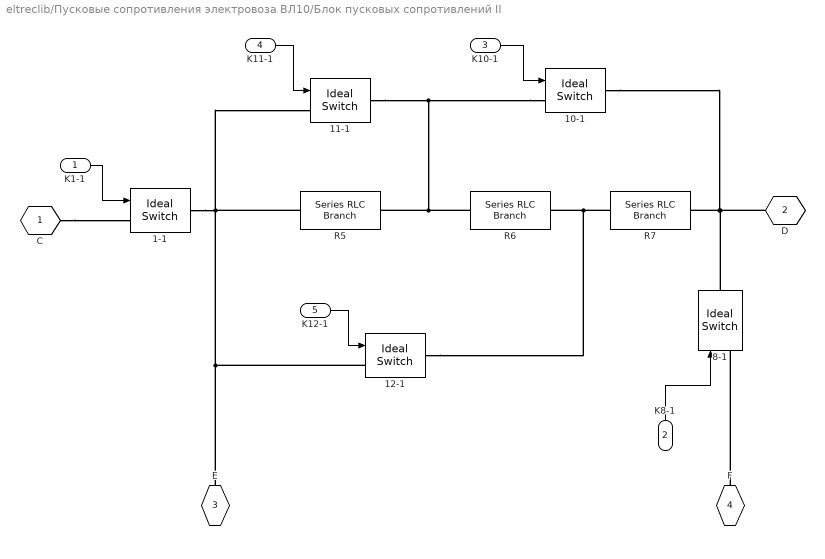
== system eltreclib/Пусковые сопротивления электровоза ВЛ10/Блок пусковых сопротивлений II ==
  K1-1 : Inport
  K8-1 : Inport  Port=2
  K10-1 : Inport  Port=3
  K11-1 : Inport  Port=4
  K12-1 : Inport  Port=5
  1-1 : powerlib/Power Electronics/Ideal Switch  Ron=0.001  Lon=0  IC=0  Rs=1e6  Cs=inf  Measurements=off
  10-1 : powerlib/Power Electronics/Ideal Switch  Ron=0.001  Lon=0  IC=0  Rs=1e6  Cs=inf  Measurements=off
  11-1 : powerlib/Power Electronics/Ideal Switch  Ron=0.001  Lon=0  IC=0  Rs=1e6  Cs=inf  Measurements=off
  12-1 : powerlib/Power Electronics/Ideal Switch  Ron=0.001  Lon=0  IC=0  Rs=1e6  Cs=inf  Measurements=off
  8-1 : powerlib/Power Electronics/Ideal Switch  Ron=0.001  Lon=0  IC=0  Rs=1e6  Cs=inf  Measurements=off
  R5 : powerlib/Elements/Series RLC Branch  LConnTagsString=__new0  RConnTagsString=__new0  BranchType=R  Resistance=4.725  Inductance=1e-3  SetiL0=off  InitialCurrent=0  Capacitance=1e-6  Setx0=off  InitialVoltage=0  Measurements=None
  R6 : powerlib/Elements/Series RLC Branch  LConnTagsString=__new0  RConnTagsString=__new0  BranchType=R  Resistance=0.841  Inductance=1e-3  SetiL0=off  InitialCurrent=0  Capacitance=1e-6  Setx0=off  InitialVoltage=0  Measurements=None
  R7 : powerlib/Elements/Series RLC Branch  LConnTagsString=__new0  RConnTagsString=__new0  BranchType=R  Resistance=1.312  Inductance=1e-3  SetiL0=off  InitialCurrent=0  Capacitance=1e-6  Setx0=off  InitialVoltage=0  Measurements=None
  C : PMIOPort  Tag=PMCPort  Port=1  Side=Left
  D : PMIOPort  Tag=PMCPort  Port=2  Side=Right
  E : PMIOPort  Tag=PMCPort  Port=3  Side=Left
  F : PMIOPort  Tag=PMCPort  Port=4  Side=Right
  wires:
  K8-1/1 -> 8-1/1
  K11-1/1 -> 11-1/1
  K10-1/1 -> 10-1/1
  K1-1/1 -> 1-1/1
  K12-1/1 -> 12-1/1
  connections:
  F/RConn1 -- 8-1/LConn1
  10-1/LConn1 -- 11-1/RConn1 -- R5/RConn1 -- R6/LConn1
  D/RConn1 -- 8-1/RConn1 -- R7/RConn1 -- 10-1/RConn1
  12-1/RConn1 -- R7/LConn1 -- R6/RConn1
  12-1/LConn1 -- E/RConn1 -- R5/LConn1 -- 11-1/LConn1 -- 1-1/RConn1
  C/RConn1 -- 1-1/LConn1

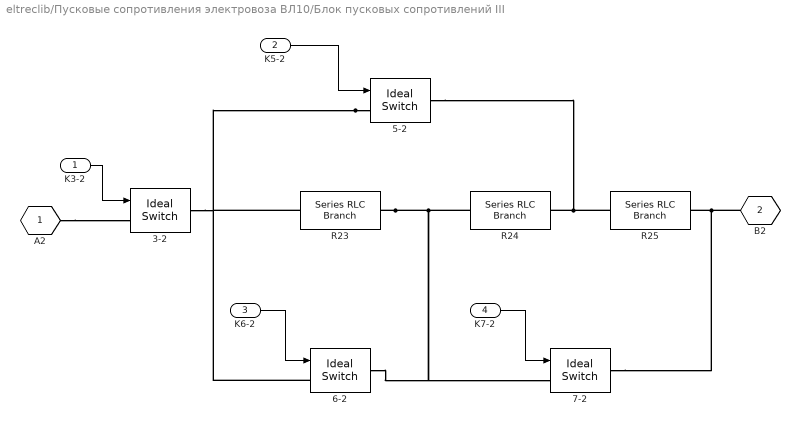
== system eltreclib/Пусковые сопротивления электровоза ВЛ10/Блок пусковых сопротивлений III ==
  K3-2 : Inport
  K5-2 : Inport  Port=2
  K6-2 : Inport  Port=3
  K7-2 : Inport  Port=4
  3-2 : powerlib/Power Electronics/Ideal Switch  Ron=0.001  Lon=0  IC=0  Rs=1e6  Cs=inf  Measurements=off
  5-2 : powerlib/Power Electronics/Ideal Switch  Ron=0.001  Lon=0  IC=0  Rs=1e6  Cs=inf  Measurements=off
  6-2 : powerlib/Power Electronics/Ideal Switch  Ron=0.001  Lon=0  IC=0  Rs=1e6  Cs=inf  Measurements=off
  7-2 : powerlib/Power Electronics/Ideal Switch  Ron=0.001  Lon=0  IC=0  Rs=1e6  Cs=inf  Measurements=off
  R23 : powerlib/Elements/Series RLC Branch  LConnTagsString=__new0  RConnTagsString=__new0  BranchType=R  Resistance=1.9425  Inductance=1e-3  SetiL0=off  InitialCurrent=0  Capacitance=1e-6  Setx0=off  InitialVoltage=0  Measurements=None
  R24 : powerlib/Elements/Series RLC Branch  LConnTagsString=__new0  RConnTagsString=__new0  BranchType=R  Resistance=0.8  Inductance=1e-3  SetiL0=off  InitialCurrent=0  Capacitance=1e-6  Setx0=off  InitialVoltage=0  Measurements=None
  R25 : powerlib/Elements/Series RLC Branch  LConnTagsString=__new0  RConnTagsString=__new0  BranchType=R  Resistance=0.61  Inductance=1e-3  SetiL0=off  InitialCurrent=0  Capacitance=1e-6  Setx0=off  InitialVoltage=0  Measurements=None
  A2 : PMIOPort  Tag=PMCPort  Port=1  Side=Left
  B2 : PMIOPort  Tag=PMCPort  Port=2  Side=Right
  wires:
  K5-2/1 -> 5-2/1
  K7-2/1 -> 7-2/1
  K3-2/1 -> 3-2/1
  K6-2/1 -> 6-2/1
  connections:
  R23/RConn1 -- R24/LConn1 -- 6-2/RConn1 -- 7-2/LConn1
  7-2/RConn1 -- R25/RConn1 -- B2/RConn1
  5-2/RConn1 -- R24/RConn1 -- R25/LConn1
  5-2/LConn1 -- 3-2/RConn1 -- R23/LConn1 -- 6-2/LConn1
  A2/RConn1 -- 3-2/LConn1

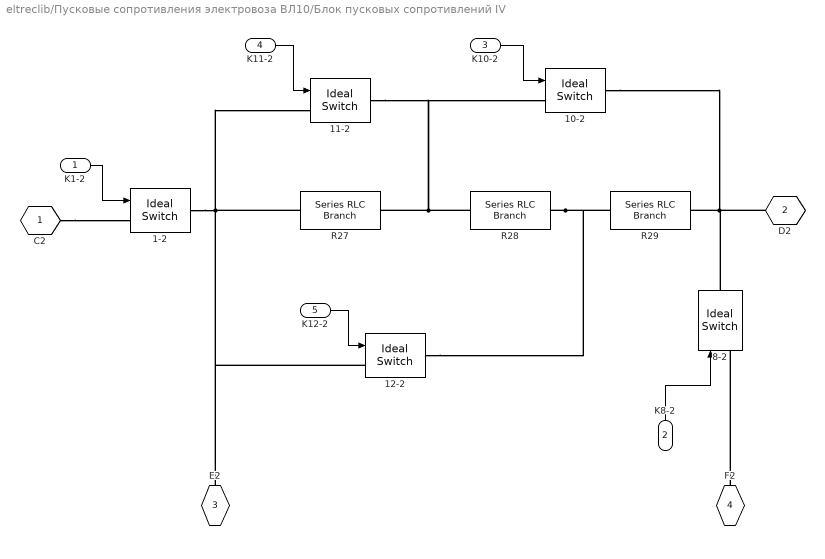
== system eltreclib/Пусковые сопротивления электровоза ВЛ10/Блок пусковых сопротивлений IV ==
  K1-2 : Inport
  K8-2 : Inport  Port=2
  K10-2 : Inport  Port=3
  K11-2 : Inport  Port=4
  K12-2 : Inport  Port=5
  1-2 : powerlib/Power Electronics/Ideal Switch  Ron=0.001  Lon=0  IC=0  Rs=1e6  Cs=inf  Measurements=off
  10-2 : powerlib/Power Electronics/Ideal Switch  Ron=0.001  Lon=0  IC=0  Rs=1e6  Cs=inf  Measurements=off
  11-2 : powerlib/Power Electronics/Ideal Switch  Ron=0.001  Lon=0  IC=0  Rs=1e6  Cs=inf  Measurements=off
  12-2 : powerlib/Power Electronics/Ideal Switch  Ron=0.001  Lon=0  IC=0  Rs=1e6  Cs=inf  Measurements=off
  8-2 : powerlib/Power Electronics/Ideal Switch  Ron=0.001  Lon=0  IC=0  Rs=1e6  Cs=inf  Measurements=off
  R27 : powerlib/Elements/Series RLC Branch  LConnTagsString=__new0  RConnTagsString=__new0  BranchType=R  Resistance=5.775  Inductance=1e-3  SetiL0=off  InitialCurrent=0  Capacitance=1e-6  Setx0=off  InitialVoltage=0  Measurements=None
  R28 : powerlib/Elements/Series RLC Branch  LConnTagsString=__new0  RConnTagsString=__new0  BranchType=R  Resistance=0.595  Inductance=1e-3  SetiL0=off  InitialCurrent=0  Capacitance=1e-6  Setx0=off  InitialVoltage=0  Measurements=None
  R29 : powerlib/Elements/Series RLC Branch  LConnTagsString=__new0  RConnTagsString=__new0  BranchType=R  Resistance=0.4315  Inductance=1e-3  SetiL0=off  InitialCurrent=0  Capacitance=1e-6  Setx0=off  InitialVoltage=0  Measurements=None
  C2 : PMIOPort  Tag=PMCPort  Port=1  Side=Left
  D2 : PMIOPort  Tag=PMCPort  Port=2  Side=Right
  E2 : PMIOPort  Tag=PMCPort  Port=3  Side=Left
  F2 : PMIOPort  Tag=PMCPort  Port=4  Side=Right
  wires:
  K12-2/1 -> 12-2/1
  K1-2/1 -> 1-2/1
  K10-2/1 -> 10-2/1
  K11-2/1 -> 11-2/1
  K8-2/1 -> 8-2/1
  connections:
  C2/RConn1 -- 1-2/LConn1
  1-2/RConn1 -- 11-2/LConn1 -- R27/LConn1 -- E2/RConn1 -- 12-2/LConn1
  R28/RConn1 -- R29/LConn1 -- 12-2/RConn1
  10-2/RConn1 -- R29/RConn1 -- 8-2/RConn1 -- D2/RConn1
  R28/LConn1 -- R27/RConn1 -- 11-2/RConn1 -- 10-2/LConn1
  F2/RConn1 -- 8-2/LConn1
